simulink model "SensorSimulinkVehicleAll"  (R2024a)
settings: Solver=FixedStepAuto  StartTime=0  StopTime=1000  FixedStep=simStepSize  RelTol=1e-3
PreLoadFcn:
  | % To support Reader and Writer blocks, some bus objects must be loaded
  | loadRoadRunnerBusObject();
undefined symbols (not defined in the file or in its folder): Defined, driving, Ego, gainArg, Lane, matlabshared, simStepSize, User
libraries: roadrunnerscenario x4, drivingscenarioandsensors x3
settings Model: Creator=The MathWorks, Inc.  LastModifiedBy=fukuchi
settings SolverCC: MaxZcPerStep=1
settings DataIOCC: SaveOutput=off  DSMLogging=off  SaveTime=off  ReturnWorkspaceOutputs=off
settings ModelReferenceCC: EnableRefExpFcnMdlSchedulingChecks=on
settings RTWCC: GPUComputeCapability=3.5  DLArmComputeVersion=19.05

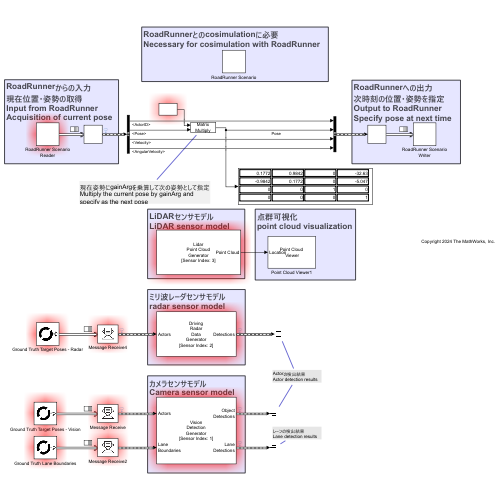
[thumbnail: Simulink's stored preview of the top-level diagram]
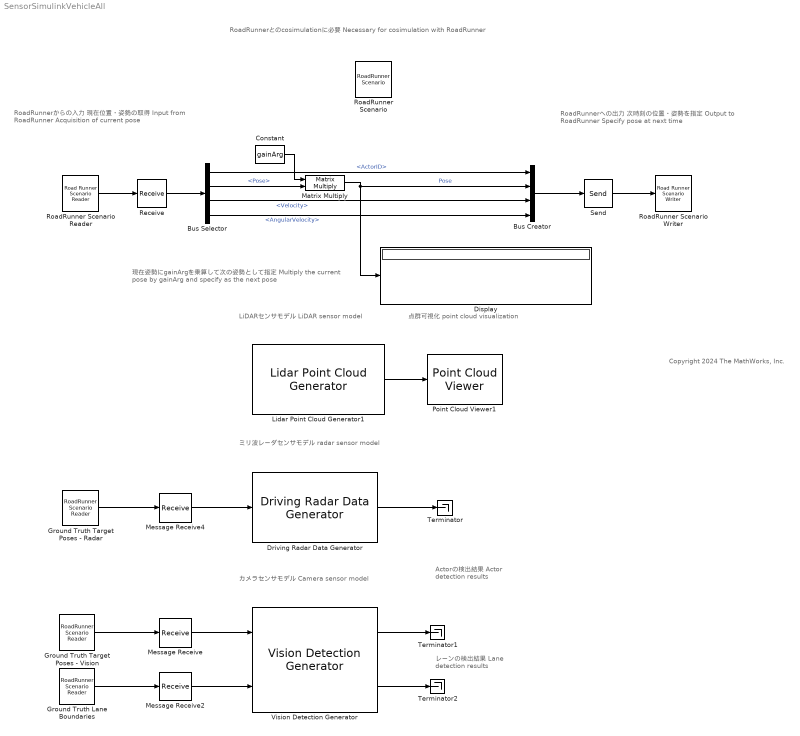
== system SensorSimulinkVehicleAll ==
  note: Copyright 2024 The MathWorks, Inc.
  note: カメラセンサモデル
      | Camera sensor model
  note: Actorの検出結果
      | Actor detection results
  note: レーンの検出結果
      | Lane detection results
  note: ミリ波レーダセンサモデル
      | radar sensor model
  note: LiDARセンサモデル
      | LiDAR sensor model
  note: 点群可視化
      | point cloud visualization
  note: RoadRunnerからの入力
      | 現在位置・姿勢の取得
      | Input from RoadRunner
      | Acquisition of current pose
  note: 現在姿勢にgainArgを乗算して次の姿勢として指定
      | Multiply the current pose by gainArg and specify as the next pose
  note: RoadRunnerへの出力
      | 次時刻の位置・姿勢を指定
      | Output to RoadRunner
      | Specify pose at next time
  note: RoadRunnerとのcosimulationに必要
      | Necessary for cosimulation with RoadRunner
  Bus Creator : BusCreator  Inputs=4  OutDataTypeStr=Bus: BusActorRuntime  NonVirtualBus=on
  Bus Selector : BusSelector  OutputSignals=ActorID,Pose,Velocity,AngularVelocity
  Constant : Constant  Value=gainArg  VectorParams1D=off
  Display : Display
  Driving Radar Data Generator : drivingscenarioandsensors/Driving Radar Data Generator  SensorIndex=2  UpdateRate=1/simStepSize  MountingLocation=[1.8, 0, 0.2 ]  MountingAngles=[0 0 0]  HasElevation=off  HasRangeRate=on  HasNoise=on  HasFalseAlarms=on  HasOcclusion=on  MaxNumReportsSource=Property  MaxNumReports=10  TargetReportFormat=Detections  DetectionCoordinates=Body  TrackCoordinates=Body  BusNameSource=Auto  BusName=BusDrivingRadarDataGenerator  AzimuthResolution=1  ElevationResolution=5  RangeResolution=2.5  RangeRateResolution=0.5  AzimuthBiasFraction=0.1  ElevationBiasFraction=0.1  RangeBiasFraction=0.05  RangeRateBiasFraction=0.05  FieldOfView=[ 80, 5 ]  RangeLimits=[ 0, 150 ]  RangeRateLimits=[ -100, 100 ]  DetectionProbability=0.9  FalseAlarmRate=1e-06  ReferenceRange=100  ReferenceRCS=0  CenterFrequency=77e9  FilterInitializationFcn=initcvekf  ConfirmationThreshold=[2 3]  DeletionThreshold=[5 5]  InitialSeedSource=Repeatable  InitialSeed=0  UsedSeed=matlabshared.tracking.internal.SimulinkUtilities.seedManager(gcb)  ProfilesSource=From Scenario Reader block  ProfilesParameters=driving.internal.ActorProfilesRadarParameters  ProfilesExpression=struct('ClassID',0,'Length',4.7,'Width',1.8,'Height',1.4,'OriginOffset',[-1.35 0 0],'RCSPattern',[10 10;10 10],'RCSAzimuthAngles',[-180 180],'RCSElevationAngles',[-90 90])
  Ground Truth Lane Boundaries : roadrunnerscenario/RoadRunner Scenario Reader  TopicCategory=Sensor  ActorCategory=All Types  ActionType=Path Following  EventType=User-Defined  TopicType=Actor Pose  VehicleType=Vehicle Pose  UserDefinedAction=Action1  UserDefinedEvent=Event1  Filter=Self  SensorTopic=Lane Boundaries  LaneBoundaryOutputTopic=All Lanes  SensorID=1  SampleTime=simStepSize
  Ground Truth Target Poses - Radar : roadrunnerscenario/RoadRunner Scenario Reader  TopicCategory=Sensor  ActorCategory=All Types  ActionType=Path Following  EventType=User-Defined  TopicType=Actor Specifications  VehicleType=Vehicle Specifications  UserDefinedAction=Action1  UserDefinedEvent=Event1  Filter=Self  SensorTopic=Target Poses  LaneBoundaryOutputTopic=Ego-Lane  SensorID=2  SampleTime=simStepSize
  Ground Truth Target Poses - Vision : roadrunnerscenario/RoadRunner Scenario Reader  TopicCategory=Sensor  ActorCategory=All Types  ActionType=Path Following  EventType=User-Defined  TopicType=Actor Specifications  VehicleType=Vehicle Specifications  UserDefinedAction=Action1  UserDefinedEvent=Event1  Filter=Self  SensorTopic=Target Poses  LaneBoundaryOutputTopic=Ego-Lane  SensorID=1  SampleTime=simStepSize
  Lidar Point Cloud Generator1 : drivingscenarioandsensors/Lidar Point Cloud Generator  SensorIndex=3  UpdateInterval=simStepSize  SensorLocation=[1.5 0]  Height=1.6  Yaw=0  Pitch=0  Roll=0  DetectionCoordinates=Ego Cartesian  HasEgoVehicle=on  EgoVehicleActorID=2  HasRoadsInputPort=on  ActorProfilesSource=From Scenario Reader block  ActorProfilesVariableName=actor_profiles  MaxRange=120  RangeAccuracy=0.002  AzimuthResolution=0.16  ElevationResolution=1.25  AzimuthLimits=[ -180, 180 ]  ElevationLimits=[ -20, 20 ]  HasNoise=on
  Matrix Multiply : Product  Multiplication=Matrix(*)
  Message Receive : Receive  InputPortMessageModes=m  UseInternalQueue=off  SampleTime=simStepSize
  Message Receive2 : Receive  InputPortMessageModes=m  UseInternalQueue=off  SampleTime=simStepSize
  Message Receive4 : Receive  InputPortMessageModes=m  UseInternalQueue=off  SampleTime=simStepSize
  Point Cloud Viewer1 : PointCloudViewer  FigPos=[661 707 598.4 335.2]
  Receive : Receive  InputPortMessageModes=m  UseInternalQueue=off  QueueOverwriting=on  QueueLength=1  QueueType=LIFO
  RoadRunner Scenario : roadrunnerscenario/RoadRunner Scenario  UserDefinedActions={}  UserDefinedEvents={}
  RoadRunner Scenario Reader : RoadRunnerScenarioReader  OutputPortMessageModes=m  TopicType=Actor Pose  VehicleType=Vehicle Specifications  SampleTime=simStepSize
  RoadRunner Scenario Writer : RoadRunnerScenarioWriter  InputPortMessageModes=m  TopicType=Actor Pose  VehicleType=Vehicle Pose
  Send : Send  OutputPortMessageModes=m
  Terminator : Terminator
  Terminator1 : Terminator
  Terminator2 : Terminator
  Vision Detection Generator : drivingscenarioandsensors/Vision Detection Generator  SensorIndex=1  DetectorOutput=Lanes and objects  UpdateInterval=simStepSize  LaneUpdateInterval=simStepSize  SensorLocation=[1.2 0]  Height=1.1  Yaw=0  Pitch=1  Roll=0  BusNameSource=Auto  BusName=BusObjectDetections  BusName2Source=Auto  BusName2=BusLaneDetections  MaxNumDetectionsSource=Property  MaxNumDetections=10  MaxNumLanesSource=Property  MaxNumLanes=10  DetectionCoordinates=Ego Cartesian  SimulateUsing=Interpreted execution  MaxRange=150  BoundingBoxAccuracy=5  ProcessNoiseIntensity=5  MaxSpeed=100  MaxAllowedOcclusion=0.5  MinObjectImageSize=[ 15, 15 ]  DetectionProbability=0.9  FalsePositivesPerImage=0.1  MinLaneImageSize=[ 20, 3 ]  LaneBoundaryAccuracy=3  HasNoise=on  InitialSeedSource=Repeatable  InitialSeed=0  UsedSeed=driving.internal.SimulinkUtilities.seedManager(gcb)  ActorProfilesSource=From Scenario Reader block  ActorProfilesParameters=driving.internal.ActorProfilesParameters  ActorProfilesExpression=actorProfiles  Intrinsics=driving.internal.cameraIntrinsics('FocalLength',[ 1200, 1200 ])
  wires:
  Message Receive2/1 -> Vision Detection Generator/2
  Ground Truth Target Poses - Vision/1 -> Message Receive/1
  Driving Radar Data Generator/1 -> Terminator/1
  Message Receive/1 -> Vision Detection Generator/1
  Vision Detection Generator/1 -> Terminator1/1
  Message Receive4/1 -> Driving Radar Data Generator/1
  Ground Truth Target Poses - Radar/1 -> Message Receive4/1
  Ground Truth Lane Boundaries/1 -> Message Receive2/1
  Vision Detection Generator/2 -> Terminator2/1
  Lidar Point Cloud Generator1/1 -> Point Cloud Viewer1/1
  Bus Creator/1 -> Send/1
  Constant/1 -> Matrix Multiply/1
  Bus Selector/3 -> Bus Creator/3  "<Velocity>"
  Bus Selector/4 -> Bus Creator/4  "<AngularVelocity>"
  Matrix Multiply/1 -> Bus Creator/2, Display/1  "Pose"
  Bus Selector/1 -> Bus Creator/1  "<ActorID>"
  Bus Selector/2 -> Matrix Multiply/2  "<Pose>"
  RoadRunner Scenario Reader/1 -> Receive/1
  Receive/1 -> Bus Selector/1
  Send/1 -> RoadRunner Scenario Writer/1
